simulink model "twoBodySim"  (R2014a)
settings: Solver=ode45  StartTime=0.0  StopTime=Tsim  MaxStep=1e4  RelTol=1e-3
values from neighbouring files (symbols this model uses):
  fixPositionOfMass1 = 1    [script02_simulate_earths_orbit.m]    (also in script03_simulate_eccentric_orbit.m; script04_twoEqualMassObjects.m = 0; script05_plutoAndCharon.m = 0; script06_threeBodySim.m = 0)
  G = 6.674e-11    [calcTwoBodyPlaneDynamics.m]    (also in script02_simulate_earths_orbit.m; script03_simulate_eccentric_orbit.m; script04_twoEqualMassObjects.m; script05_plutoAndCharon.m)
  m1 = 2e30    (= 2e+30)    [script02_simulate_earths_orbit.m]    (also in script03_simulate_eccentric_orbit.m; script04_twoEqualMassObjects.m = 1e+22; script05_plutoAndCharon.m = 1.3e+22; script06_threeBodySim.m = 1.3e+22)
  m2 = 1    [script02_simulate_earths_orbit.m]    (also in script03_simulate_eccentric_orbit.m; script04_twoEqualMassObjects.m = 1e+22; script05_plutoAndCharon.m = 1.5e+21; script06_threeBodySim.m = 1.5e+21)
  r1_init = -r2_init*1e-6    [script02_simulate_earths_orbit.m]    (also in script03_simulate_eccentric_orbit.m; script04_twoEqualMassObjects.m = -r2_init; script05_plutoAndCharon.m = r1; script06_threeBodySim.m = r1)
  r1dot_init = -r2dot_init*1e-6    [script02_simulate_earths_orbit.m]    (also in script03_simulate_eccentric_orbit.m; script04_twoEqualMassObjects.m = -r2dot_init; script05_plutoAndCharon.m = r1dot; script06_threeBodySim.m = r1dot)
  r2_init = [149e9 0, 0]'    [script02_simulate_earths_orbit.m]    (also in script03_simulate_eccentric_orbit.m; script04_twoEqualMassObjects.m = [1e8 0, 0]'; script05_plutoAndCharon.m = r2; script06_threeBodySim.m = r2)
  r2dot_init = [0, 29.78e3,0]'    [script02_simulate_earths_orbit.m]    (also in script03_simulate_eccentric_orbit.m = [0, 29.78e3*0.5,0]'; script04_twoEqualMassObjects.m = [0, sqrt(G*m1/(4*r2_init(1)))*0.5,0]'; script05_plutoAndCharon.m = r2dot; script06_threeBodySim.m = r2dot)
libraries: simulink x1
settings Model: Creator=Timo  LastModifiedBy=Timo

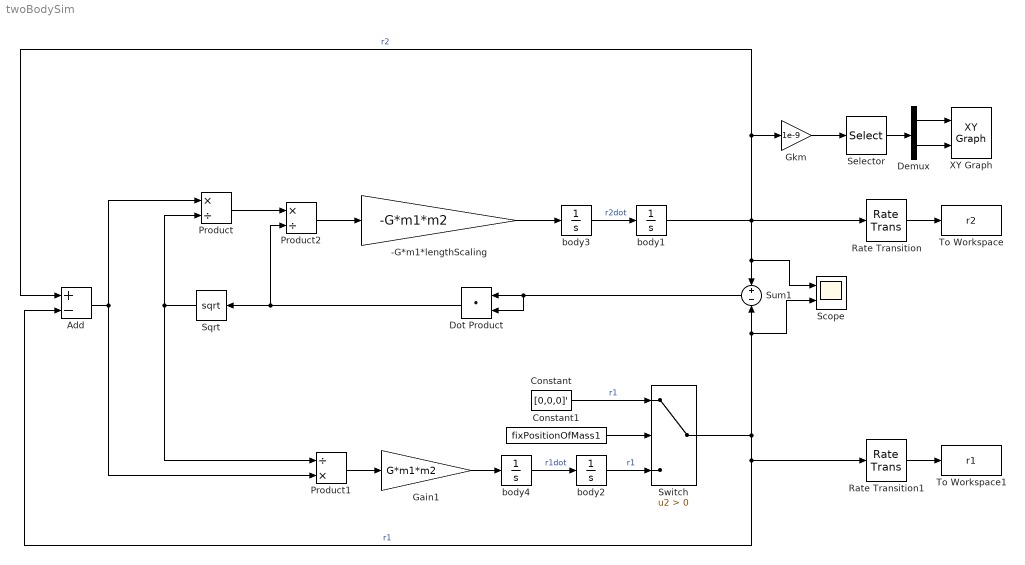
== system twoBodySim ==
  -G*m1*lengthScaling : Gain  Gain=-G*m1*m2
  Add : Sum  Inputs=+-
  Constant : Constant  Value=[0,0,0]'
  Constant1 : Constant  Value=fixPositionOfMass1
  Demux : Demux  Outputs=2
  Dot Product : DotProduct  InputSameDT=on  OutDataTypeStr=Inherit: Inherit via internal rule
  Gain1 : Gain  Gain=G*m1*m2
  Gkm : Gain  Gain=1e-9
  Product : Product  Inputs=*/
  Product1 : Product  Inputs=/*
  Product2 : Product  Inputs=*/
  Rate Transition : RateTransition  OutPortSampleTime=T_sample
  Rate Transition1 : RateTransition  OutPortSampleTime=T_sample
  Scope : Scope  NumInputPorts=2
      settings: YMin=-8.5e+14~-1  YMax=3e+14~1
  Selector : Selector  InputPortWidth=3  Indices=[1 2]
  Sqrt : Sqrt  SaturateOnIntegerOverflow=on
  Sum1 : Sum  Inputs=+-
  Switch : Switch  Criteria=u2 > Threshold
  To Workspace : ToWorkspace  VariableName=r2  SaveFormat=Timeseries  SampleTime=-1
  To Workspace1 : ToWorkspace  VariableName=r1  SaveFormat=Timeseries  SampleTime=-1
  XY Graph : simulink/Sinks/XY Graph  xmin=-2e2  xmax=2e2  ymin=-2e2  ymax=2e2  st=-1
  body1 : Integrator  InitialCondition=r2_init
  body2 : Integrator  InitialCondition=r1_init
  body3 : Integrator  InitialCondition=r2dot_init
  body4 : Integrator  InitialCondition=r1dot_init
  wires:
  body3/1 -> body1/1  "r2dot"
  body4/1 -> body2/1  "r1dot"
  -G*m1*lengthScaling/1 -> body3/1
  Switch/1 -> Scope/2, Sum1/2, Rate Transition1/1, Add/2  "r1"
  Product1/1 -> Gain1/1
  Gain1/1 -> body4/1
  body1/1 -> Add/1, Gkm/1, Rate Transition/1, Scope/1, Sum1/1  "r2"
  Demux/1 -> XY Graph/1
  Demux/2 -> XY Graph/2
  Add/1 -> Product/1, Product1/2
  Sqrt/1 -> Product/2, Product1/1
  Product2/1 -> -G*m1*lengthScaling/1
  Product/1 -> Product2/1
  Dot Product/1 -> Sqrt/1, Product2/2
  Selector/1 -> Demux/1
  Sum1/1 -> Dot Product/2, Dot Product/1
  Gkm/1 -> Selector/1
  body2/1 -> Switch/3  "r1"
  Constant/1 -> Switch/1  "r1"
  Rate Transition/1 -> To Workspace/1
  Rate Transition1/1 -> To Workspace1/1
  Constant1/1 -> Switch/2
